simulink model "position"  (R2016b)
settings: Solver=VariableStepAuto  StartTime=0.0  StopTime=1  RelTol=1e-3
model workspace (MAT data in the model file):
  TL = 0
  Ti = 0.001
  fpwm = 5000
  ts = 5e-06
undefined symbols (not defined in the file): Kii, Kiw, Kpi, Kpw, pmsm, Ts, Tw
libraries: nesl_utility x13, fl_lib x10, simulink x6, pe_lib x4, pePwmGeneratorTwoLevel x1
settings Model: Creator=25097  LastModifiedBy=25097

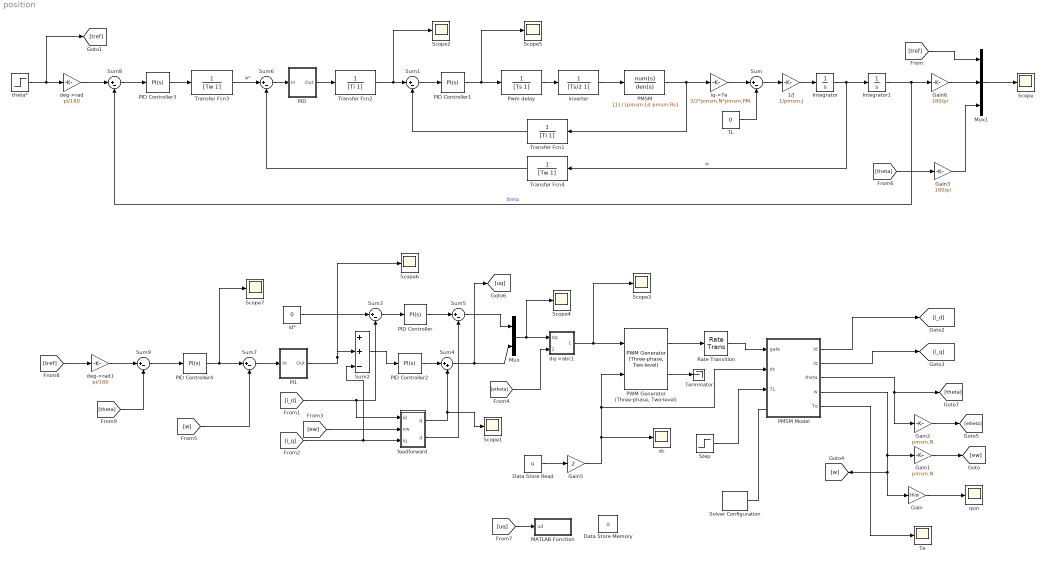
== system position ==
  1/J : Gain  Gain=1/pmsm.J
  Data Store Memory : DataStoreMemory  DataStoreName=u  ReadBeforeWriteMsg=warning  WriteAfterWriteMsg=warning  WriteAfterReadMsg=warning  InitialValue=10  ShowAdditionalParam=off  OutDataTypeStr=double
  Data Store Read : DataStoreRead  DataStoreName=u  DataStoreElements=u
  Gain : Gain  Gain=30/pi
  Gain1 : Gain  Gain=pmsm.N
  Gain2 : Gain  Gain=pmsm.N
  Gain3 : Gain  Gain=180/pi
  Gain5 : Gain  Gain=2
  Gain6 : Gain  Gain=180/pi
  Integrator : Integrator
  Integrator1 : Integrator
  MATLAB Function : MATLAB Function  TreatAsAtomicUnit=on
  Mux : Mux  Inputs=2
  Mux1 : Mux  Inputs=3
  PI1 : Subsystem
  PID : Subsystem
  PID Controller : simulink/Continuous/PID Controller  Controller=PI  TimeDomain=Continuous-time  SampleTime=-1  IntegratorMethod=Forward Euler  FilterMethod=Forward Euler  Form=Parallel  UseFilter=on  ControllerParametersSource=internal  P=Kpi  I=Kii  D=0  N=100  InitialConditionSource=internal  InitialConditionForIntegrator=0  InitialConditionForFilter=0  ExternalReset=none  LimitOutput=off  UpperSaturationLimit=inf  LowerSaturationLimit=-inf  LinearizeAsGain=on  AntiWindupMode=none  Kb=1  TrackingMode=off  Kt=1  PParamMin=[]  PParamMax=[]  IParamMin=[]  IParamMax=[]  DParamMin=[]  DParamMax=[]  NParamMin=[]  NParamMax=[]  KbParamMin=[]  KbParamMax=[]  KtParamMin=[]  KtParamMax=[]  POutMin=[]  POutMax=[]  IOutMin=[]  IOutMax=[]  DOutMin=[]  DOutMax=[]  NOutMin=[]  NOutMax=[]  KbOutMin=[]  KbOutMax=[]  KtOutMin=[]  KtOutMax=[]  IntegratorOutMin=[]  IntegratorOutMax=[]  FilterOutMin=[]  FilterOutMax=[]  SumOutMin=[]  SumOutMax=[]  SumI1OutMin=[]  SumI1OutMax=[]  SumI2OutMin=[]  SumI2OutMax=[]  SumI3OutMin=[]  SumI3OutMax=[]  SumDOutMin=[]  SumDOutMax=[]  SaturationOutMin=[]  SaturationOutMax=[]  IntegratorContinuousStateAttributes=''  IntegratorStateMustResolveToSignalObject=off  IntegratorRTWStateStorageClass=Auto  FilterContinuousStateAttributes=''  FilterStateMustResolveToSignalObject=off  FilterRTWStateStorageClass=Auto  DifferentiatorICPrevScaledInput=0  DifferentiatorOutMin=[]  DifferentiatorOutMax=[]
  PID Controller1 : simulink/Continuous/PID Controller  Controller=PI  TimeDomain=Continuous-time  SampleTime=-1  IntegratorMethod=Forward Euler  FilterMethod=Forward Euler  Form=Parallel  UseFilter=on  ControllerParametersSource=internal  P=Kpi  I=Kii  D=0  N=100  InitialConditionSource=internal  InitialConditionForIntegrator=0  InitialConditionForFilter=0  ExternalReset=none  LimitOutput=off  UpperSaturationLimit=5  LowerSaturationLimit=-5  LinearizeAsGain=on  AntiWindupMode=none  Kb=1  TrackingMode=off  Kt=1  PParamMin=[]  PParamMax=[]  IParamMin=[]  IParamMax=[]  DParamMin=[]  DParamMax=[]  NParamMin=[]  NParamMax=[]  KbParamMin=[]  KbParamMax=[]  KtParamMin=[]  KtParamMax=[]  POutMin=[]  POutMax=[]  IOutMin=[]  IOutMax=[]  DOutMin=[]  DOutMax=[]  NOutMin=[]  NOutMax=[]  KbOutMin=[]  KbOutMax=[]  KtOutMin=[]  KtOutMax=[]  IntegratorOutMin=[]  IntegratorOutMax=[]  FilterOutMin=[]  FilterOutMax=[]  SumOutMin=[]  SumOutMax=[]  SumI1OutMin=[]  SumI1OutMax=[]  SumI2OutMin=[]  SumI2OutMax=[]  SumI3OutMin=[]  SumI3OutMax=[]  SumDOutMin=[]  SumDOutMax=[]  SaturationOutMin=[]  SaturationOutMax=[]  IntegratorContinuousStateAttributes=''  IntegratorStateMustResolveToSignalObject=off  IntegratorRTWStateStorageClass=Auto  FilterContinuousStateAttributes=''  FilterStateMustResolveToSignalObject=off  FilterRTWStateStorageClass=Auto  DifferentiatorICPrevScaledInput=0  DifferentiatorOutMin=[]  DifferentiatorOutMax=[]
  PID Controller2 : simulink/Continuous/PID Controller  Controller=PI  TimeDomain=Continuous-time  SampleTime=-1  IntegratorMethod=Forward Euler  FilterMethod=Forward Euler  Form=Parallel  UseFilter=on  ControllerParametersSource=internal  P=Kpi  I=Kii  D=0  N=100  InitialConditionSource=internal  InitialConditionForIntegrator=0  InitialConditionForFilter=0  ExternalReset=none  LimitOutput=off  UpperSaturationLimit=inf  LowerSaturationLimit=-inf  LinearizeAsGain=on  AntiWindupMode=none  Kb=1  TrackingMode=off  Kt=1  PParamMin=[]  PParamMax=[]  IParamMin=[]  IParamMax=[]  DParamMin=[]  DParamMax=[]  NParamMin=[]  NParamMax=[]  KbParamMin=[]  KbParamMax=[]  KtParamMin=[]  KtParamMax=[]  POutMin=[]  POutMax=[]  IOutMin=[]  IOutMax=[]  DOutMin=[]  DOutMax=[]  NOutMin=[]  NOutMax=[]  KbOutMin=[]  KbOutMax=[]  KtOutMin=[]  KtOutMax=[]  IntegratorOutMin=[]  IntegratorOutMax=[]  FilterOutMin=[]  FilterOutMax=[]  SumOutMin=[]  SumOutMax=[]  SumI1OutMin=[]  SumI1OutMax=[]  SumI2OutMin=[]  SumI2OutMax=[]  SumI3OutMin=[]  SumI3OutMax=[]  SumDOutMin=[]  SumDOutMax=[]  SaturationOutMin=[]  SaturationOutMax=[]  IntegratorContinuousStateAttributes=''  IntegratorStateMustResolveToSignalObject=off  IntegratorRTWStateStorageClass=Auto  FilterContinuousStateAttributes=''  FilterStateMustResolveToSignalObject=off  FilterRTWStateStorageClass=Auto  DifferentiatorICPrevScaledInput=0  DifferentiatorOutMin=[]  DifferentiatorOutMax=[]
  PID Controller3 : simulink/Continuous/PID Controller  Controller=PI  TimeDomain=Continuous-time  SampleTime=-1  IntegratorMethod=Forward Euler  FilterMethod=Forward Euler  Form=Parallel  UseFilter=on  ControllerParametersSource=internal  P=19  I=8.8  D=0  N=100  InitialConditionSource=internal  InitialConditionForIntegrator=0  InitialConditionForFilter=0  ExternalReset=none  LimitOutput=off  UpperSaturationLimit=inf  LowerSaturationLimit=-inf  LinearizeAsGain=on  AntiWindupMode=none  Kb=1  TrackingMode=off  Kt=1  PParamMin=[]  PParamMax=[]  IParamMin=[]  IParamMax=[]  DParamMin=[]  DParamMax=[]  NParamMin=[]  NParamMax=[]  KbParamMin=[]  KbParamMax=[]  KtParamMin=[]  KtParamMax=[]  POutMin=[]  POutMax=[]  IOutMin=[]  IOutMax=[]  DOutMin=[]  DOutMax=[]  NOutMin=[]  NOutMax=[]  KbOutMin=[]  KbOutMax=[]  KtOutMin=[]  KtOutMax=[]  IntegratorOutMin=[]  IntegratorOutMax=[]  FilterOutMin=[]  FilterOutMax=[]  SumOutMin=[]  SumOutMax=[]  SumI1OutMin=[]  SumI1OutMax=[]  SumI2OutMin=[]  SumI2OutMax=[]  SumI3OutMin=[]  SumI3OutMax=[]  SumDOutMin=[]  SumDOutMax=[]  SaturationOutMin=[]  SaturationOutMax=[]  IntegratorContinuousStateAttributes=''  IntegratorStateMustResolveToSignalObject=off  IntegratorRTWStateStorageClass=Auto  FilterContinuousStateAttributes=''  FilterStateMustResolveToSignalObject=off  FilterRTWStateStorageClass=Auto  DifferentiatorICPrevScaledInput=0  DifferentiatorOutMin=[]  DifferentiatorOutMax=[]
  PID Controller4 : simulink/Continuous/PID Controller  Controller=PI  TimeDomain=Continuous-time  SampleTime=-1  IntegratorMethod=Forward Euler  FilterMethod=Forward Euler  Form=Parallel  UseFilter=on  ControllerParametersSource=internal  P=19  I=20  D=0  N=100  InitialConditionSource=internal  InitialConditionForIntegrator=0  InitialConditionForFilter=0  ExternalReset=none  LimitOutput=off  UpperSaturationLimit=inf  LowerSaturationLimit=-inf  LinearizeAsGain=on  AntiWindupMode=none  Kb=1  TrackingMode=off  Kt=1  PParamMin=[]  PParamMax=[]  IParamMin=[]  IParamMax=[]  DParamMin=[]  DParamMax=[]  NParamMin=[]  NParamMax=[]  KbParamMin=[]  KbParamMax=[]  KtParamMin=[]  KtParamMax=[]  POutMin=[]  POutMax=[]  IOutMin=[]  IOutMax=[]  DOutMin=[]  DOutMax=[]  NOutMin=[]  NOutMax=[]  KbOutMin=[]  KbOutMax=[]  KtOutMin=[]  KtOutMax=[]  IntegratorOutMin=[]  IntegratorOutMax=[]  FilterOutMin=[]  FilterOutMax=[]  SumOutMin=[]  SumOutMax=[]  SumI1OutMin=[]  SumI1OutMax=[]  SumI2OutMin=[]  SumI2OutMax=[]  SumI3OutMin=[]  SumI3OutMax=[]  SumDOutMin=[]  SumDOutMax=[]  SaturationOutMin=[]  SaturationOutMax=[]  IntegratorContinuousStateAttributes=''  IntegratorStateMustResolveToSignalObject=off  IntegratorRTWStateStorageClass=Auto  FilterContinuousStateAttributes=''  FilterStateMustResolveToSignalObject=off  FilterRTWStateStorageClass=Auto  DifferentiatorICPrevScaledInput=0  DifferentiatorOutMin=[]  DifferentiatorOutMax=[]
  "PMSM " : TransferFcn  Denominator=[pmsm.Ld pmsm.Rs]
  PMSM Model : Subsystem
      settings: MinAlgLoopOccurrences=on
  "PWM Generator (Three-phase, Two-level)" : pePwmGeneratorTwoLevel/PWM Generator (Three-phase, Two-level)  OverrideUsingVariant=NaturalMode  PWMMode=Continuous PWM (CPWM)  CPWMMode=SPWM: sinusoidal PWM  DPWMMode=60 DPWM: 60 degree discontinuous PWM  fsw=fpwm  Ts=ts
      settings: SamplingMode=Natural
  "Pwm delay " : TransferFcn  Denominator=[Ts 1]
  Rate Transition : RateTransition
  Scope{,1..7} (8 alike) : Scope
  Solver Configuration : nesl_utility/Solver Configuration  PhysicalDomain=network_engine_domain  SubClassName=solver  LeftPortType=input  RightPortType=generic  Accelerate=off  Tones=[]  Harmonics=[]  SimulateNoise=off  Profile=off  UseLocalSampling=off  EnableSwitchedLinearOptims=on  FrequencyDomain=off  UseCCode=off  RelTol=0.001  AbsTol=1e-06  MinStep=1e-09  ToWorkspace=off  RevertToSquareIcSolve=off  NumHomotopyIterations=100  PhasorMode=off  PhasorModeNumHarmonics=1  OverrideAbsTol=off  DoDC=off  ResidualTolerance=1e-07  UseLocalSolver=off  LocalSolverChoice=NE_BACKWARD_EULER_ADVANCER  LocalSolverSampleTime=1e-6  DoFixedCost=off  MaxNonlinIter=3  MaxModeIter=2  LinearAlgebra=Sparse  DelaysMemoryBudget=1024  AutomaticFiltering=on  FilteringTimeConstant=0.001
  Step : Step  Time=0.4  After=TL  SampleTime=0
  Sum{,1,3,5..9} (8 alike) : Sum  Inputs=|+-
  Sum2 : Sum  Inputs=|++-
  Sum4 : Sum  Inputs=|++
  TL : Constant  Value=0
  Te : Scope
  Terminator : Terminator
  Transfer Fcn1 : TransferFcn  Denominator=[Ti 1]
  Transfer Fcn2 : TransferFcn  Denominator=[Ti 1]
  Transfer Fcn3 : TransferFcn  Denominator=[Tw 1]
  Transfer Fcn4 : TransferFcn  Numerator=[ 1]  Denominator=[Tw 1]
  dc : Scope
  deg->rad : Gain  Gain=pi/180
  deg->rad1 : Gain  Gain=pi/180
  dq->abc1 : Subsystem
  "feedforward " : Subsystem
  id* : Constant  Value=0
  inverter : TransferFcn  Denominator=[Ts/2 1]
  iq->Te : Gain  Gain=3/2*pmsm.N*pmsm.PM
  rpm : Scope
  theta* : Step  Time=0.05  After=30  SampleTime=0
  wires:
  Transfer Fcn2/1 -> Scope2/1, Sum1/1
  Sum1/1 -> PID Controller1/1
  PID Controller1/1 -> Scope5/1, "Pwm delay "/1
  "Pwm delay "/1 -> inverter/1
  inverter/1 -> "PMSM "/1
  "PMSM "/1 -> Transfer Fcn1/1, iq->Te/1
  Transfer Fcn1/1 -> Sum1/2
  Sum2/1 -> PID Controller2/1
  PID Controller2/1 -> Sum4/1
  id*/1 -> Sum3/1
  Sum3/1 -> PID Controller/1
  PID Controller/1 -> Sum5/1
  "feedforward "/1(q) -> Sum4/2, Scope1/1
  "feedforward "/2(d) -> Sum5/2
  [ew] -> "feedforward "/2(ew)
  Sum4/1 -> [uq], Mux/2
  Sum5/1 -> Mux/1
  Mux/1 -> Scope4/1, dq->abc1/1(dq)
  [etheta] -> dq->abc1/2("theta ")
  Gain5/1 -> dc/1, "PWM Generator (Three-phase, Two-level)"/2, PMSM Model/2(dc)
  "PWM Generator (Three-phase, Two-level)"/2 -> Terminator/1
  PMSM Model/3(theta) -> Gain2/1, [theta]
  Mux1/1 -> Scope/1
  Gain/1 -> rpm/1
  PMSM Model/5("Te ") -> Te/1
  PMSM Model/4(w) -> Gain1/1, [w], Gain/1
  Gain2/1 -> [etheta]
  Gain1/1 -> [ew]
  PMSM Model/1(id) -> [i_d]
  PMSM Model/2(iq) -> [i_q]
  [i_d] -> "feedforward "/1("id "), Sum3/2
  [i_q] -> Sum2/3, "feedforward "/3(iq)
  dq->abc1/1(abc) -> Scope3/1, "PWM Generator (Three-phase, Two-level)"/1
  "PWM Generator (Three-phase, Two-level)"/1 -> Rate Transition/1
  Rate Transition/1 -> PMSM Model/1("gate ")
  iq->Te/1 -> Sum/1
  TL/1 -> Sum/2
  Sum/1 -> 1/J/1
  1/J/1 -> Integrator/1
  Integrator/1 -> Integrator1/1, Transfer Fcn4/1  "w"
  Transfer Fcn3/1 -> Sum6/1  "w*"
  Transfer Fcn4/1 -> Sum6/2
  PID Controller3/1 -> Transfer Fcn3/1
  Sum6/1 -> PID/1(In)
  PID/1(Out) -> Transfer Fcn2/1
  theta*/1 -> [tref], deg->rad/1
  Sum7/1 -> PI1/1(In)
  PI1/1(Out) -> Scope6/1, Sum2/2
  [w] -> Sum7/2
  [uq] -> MATLAB Function/1(ud)
  Data Store Read/1 -> Gain5/1
  Step/1 -> PMSM Model/3(TL)
  Integrator1/1 -> Sum8/2, Gain6/1  "theta"
  Gain6/1 -> Mux1/2
  deg->rad/1 -> Sum8/1
  Sum8/1 -> PID Controller3/1
  [tref] -> Mux1/1
  PID Controller4/1 -> Scope7/1, Sum7/1
  [tref] -> deg->rad1/1
  deg->rad1/1 -> Sum9/1
  Sum9/1 -> PID Controller4/1
  [theta] -> Sum9/2
  [theta] -> Gain3/1
  Gain3/1 -> Mux1/3
  connections:
  Solver Configuration/RConn1 -- PMSM Model/LConn1

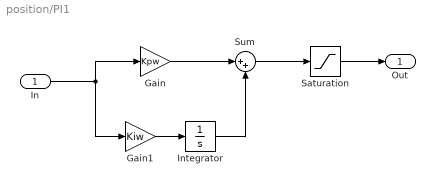
== system position/PI1 ==
  In : Inport
  Gain : Gain  Gain=Kpw
  Gain1 : Gain  Gain=Kiw
  Integrator : Integrator  LimitOutput=on  UpperSaturationLimit=pmsm.Imax*0.5  LowerSaturationLimit=-pmsm.Imax*0.5
  Saturation : Saturate  UpperLimit=pmsm.Imax  LowerLimit=-pmsm.Imax
  Sum : Sum  Inputs=|++
  Out : Outport
  wires:
  Saturation/1 -> Out/1
  Sum/1 -> Saturation/1
  Integrator/1 -> Sum/2
  Gain/1 -> Sum/1
  Gain1/1 -> Integrator/1
  In/1 -> Gain/1, Gain1/1

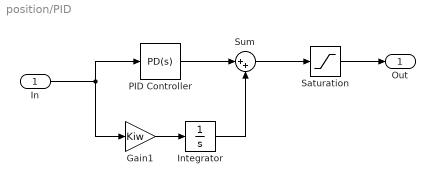
== system position/PID ==
  In : Inport
  Gain1 : Gain  Gain=Kiw
  Integrator : Integrator  LimitOutput=on  UpperSaturationLimit=pmsm.Imax*0.5  LowerSaturationLimit=-pmsm.Imax*0.5
  PID Controller : simulink/Continuous/PID Controller  Controller=PD  TimeDomain=Continuous-time  SampleTime=-1  IntegratorMethod=Forward Euler  FilterMethod=Forward Euler  Form=Parallel  UseFilter=on  ControllerParametersSource=internal  P=Kpw  I=1  D=0.01  N=100  InitialConditionSource=internal  InitialConditionForIntegrator=0  InitialConditionForFilter=0  ExternalReset=none  LimitOutput=off  UpperSaturationLimit=inf  LowerSaturationLimit=-inf  LinearizeAsGain=on  AntiWindupMode=none  Kb=1  TrackingMode=off  Kt=1  PParamMin=[]  PParamMax=[]  IParamMin=[]  IParamMax=[]  DParamMin=[]  DParamMax=[]  NParamMin=[]  NParamMax=[]  KbParamMin=[]  KbParamMax=[]  KtParamMin=[]  KtParamMax=[]  POutMin=[]  POutMax=[]  IOutMin=[]  IOutMax=[]  DOutMin=[]  DOutMax=[]  NOutMin=[]  NOutMax=[]  KbOutMin=[]  KbOutMax=[]  KtOutMin=[]  KtOutMax=[]  IntegratorOutMin=[]  IntegratorOutMax=[]  FilterOutMin=[]  FilterOutMax=[]  SumOutMin=[]  SumOutMax=[]  SumI1OutMin=[]  SumI1OutMax=[]  SumI2OutMin=[]  SumI2OutMax=[]  SumI3OutMin=[]  SumI3OutMax=[]  SumDOutMin=[]  SumDOutMax=[]  SaturationOutMin=[]  SaturationOutMax=[]  IntegratorContinuousStateAttributes=''  IntegratorStateMustResolveToSignalObject=off  IntegratorRTWStateStorageClass=Auto  FilterContinuousStateAttributes=''  FilterStateMustResolveToSignalObject=off  FilterRTWStateStorageClass=Auto  DifferentiatorICPrevScaledInput=0  DifferentiatorOutMin=[]  DifferentiatorOutMax=[]
  Saturation : Saturate  UpperLimit=pmsm.Imax  LowerLimit=-pmsm.Imax
  Sum : Sum  Inputs=|++
  Out : Outport
  wires:
  In/1 -> PID Controller/1, Gain1/1
  Gain1/1 -> Integrator/1
  PID Controller/1 -> Sum/1
  Integrator/1 -> Sum/2
  Sum/1 -> Saturation/1
  Saturation/1 -> Out/1

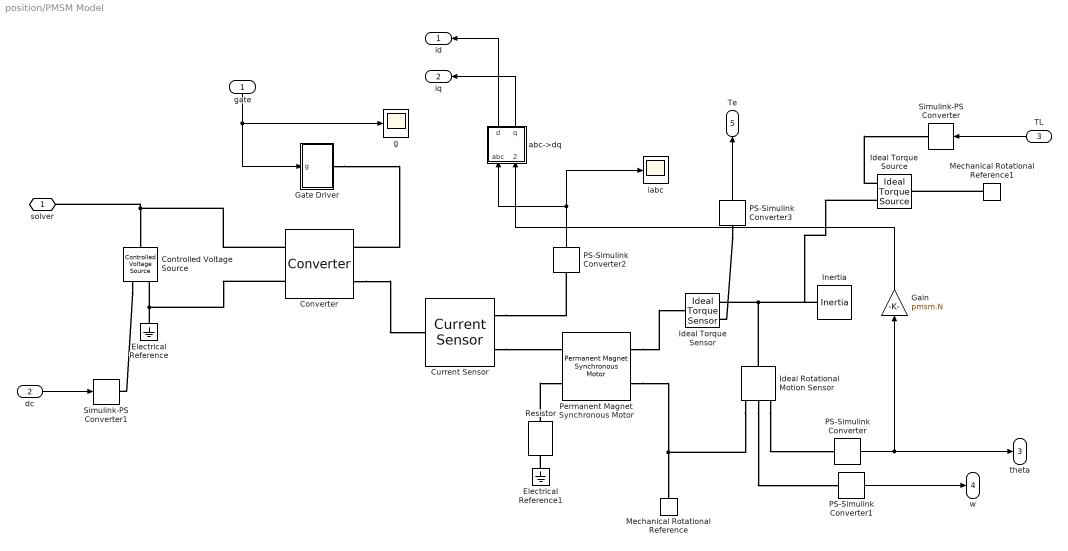
== system position/PMSM Model ==
  "gate " : Inport
  dc : Inport  Port=2
  TL : Inport  Port=3
  Controlled Voltage Source : fl_lib/Electrical/Electrical Sources/Controlled Voltage Source
  Converter : pe_lib/Semiconductors/Converter  device_type=2  Vf=0.8 V  Ron=0.001 Ohm  Rds=0.001 Ohm  Goff=1e-8 1/Ohm  Vth=0.5 V  Vgt=1 V  Vgt_off=-1 V  Ih=1 A  diode_param=1  diode_Vf=0.8 V  diode_Ron=0.001 Ohm  diode_Goff=1e-5 1/Ohm  diode_C=50 nF  diode_iRM=-235 A  diode_iF=300 A  diode_idot=-50 A/us  diode_trr_param=1  diode_trr_factor=3  diode_trr=15 us  diode_Qrr=1.5e+3 s*uA  snubber_type=0  Rs=0.1 Ohm  Cs=1e-7 F
  Current Sensor : pe_lib/Sensors/Current Sensor
  Electrical Reference : fl_lib/Electrical/Electrical Elements/Electrical Reference
  Electrical Reference1 : fl_lib/Electrical/Electrical Elements/Electrical Reference
  Gain : Gain  Gain=pmsm.N
  Gate Driver : Subsystem
  Ideal Rotational Motion Sensor : fl_lib/Mechanical/Mechanical Sensors/Ideal Rotational Motion Sensor  offset=0 rad
  Ideal Torque Sensor : fl_lib/Mechanical/Mechanical Sensors/Ideal Torque Sensor
  Ideal Torque Source : fl_lib/Mechanical/Mechanical Sources/Ideal Torque Source
  Inertia : fl_lib/Mechanical/Rotational Elements/Inertia  inertia=pmsm.J kg*m^2  w_specify=off  w_priority=High  w=0 rad/s  t_specify=off  t_priority=None  t=0 N*m
  Mechanical Rotational Reference : fl_lib/Mechanical/Rotational Elements/Mechanical Rotational Reference
  Mechanical Rotational Reference1 : fl_lib/Mechanical/Rotational Elements/Mechanical Rotational Reference
  PS-Simulink Converter{,1..3} (4 alike) : nesl_utility/PS-Simulink Converter  PhysicalDomain=network_engine_domain  SubClassName=ps_output  LeftPortType=input  RightPortType=output  PseudoPeriodic=off  Frequencies=[]  Unit=1  AffineConversion=off
  Permanent Magnet Synchronous Motor : pe_lib/Machines/Permanent Magnet Rotor/Permanent Magnet Synchronous Motor  nPolePairs=pmsm.N  pm_flux_linkage=pmsm.PM Wb  stator_param=1  Ld=pmsm.Ld H  Lq=pmsm.Ld H  L0=pmsm.Ld H  Ls=0.0002 H  Lm=0.00002 H  Ms=0.00002 H  Rs=pmsm.Rs Ohm  initial_currents=[0.0, 0.0, 0.0] A  axes_param=2  angular_position0=0 rad  rotor_offset=-pi / 2 rad  shift_3ph=[nan, nan, nan] rad  sqrt2OverSqrt3=nan  oneOverSqrt2=nan  twoPiOver3=nan  Lmin=1e-9 H
  Resistor : fl_lib/Electrical/Electrical Elements/Resistor  R=1e9 Ohm  i_specify=off  i_priority=None  i=0 A  v_specify=off  v_priority=None  v=0 V
  Simulink-PS Converter : nesl_utility/Simulink-PS Converter  PhysicalDomain=network_engine_domain  SubClassName=ps_input  LeftPortType=input  RightPortType=output  PseudoPeriodic=off  Frequencies=[]  NoiseDistribution=none  NoiseParameters=[]  Unit=1  AffineConversion=off  InputFiltering=off  SimscapeFilterOrder=1  InputFilterTimeConstant=0.001  UdotUserProvided=1
  Simulink-PS Converter1 : nesl_utility/Simulink-PS Converter  PhysicalDomain=network_engine_domain  SubClassName=ps_input  LeftPortType=input  RightPortType=output  PseudoPeriodic=off  Frequencies=[]  NoiseDistribution=none  NoiseParameters=[]  Unit=1  AffineConversion=off  InputFiltering=off  SimscapeFilterOrder=1  InputFilterTimeConstant=0.001  UdotUserProvided=1
  abc->dq : Subsystem
  g : Scope
  iabc : Scope
  "solver " : PMIOPort  Port=1  Side=Left
  id : Outport
  iq : Outport  Port=2
  theta : Outport  Port=3
  w : Outport  Port=4
  "Te " : Outport  Port=5
  wires:
  PS-Simulink Converter/1 -> Gain/1, theta/1
  PS-Simulink Converter2/1 -> abc->dq/1(abc), iabc/1
  PS-Simulink Converter1/1 -> w/1
  abc->dq/1(d) -> id/1
  abc->dq/2(q) -> iq/1
  PS-Simulink Converter3/1 -> "Te "/1
  Gain/1 -> abc->dq/2(theta)
  "gate "/1 -> g/1, Gate Driver/1(g)
  dc/1 -> Simulink-PS Converter1/1
  TL/1 -> Simulink-PS Converter/1
  connections:
  Electrical Reference/LConn1 -- Converter/RConn2 -- Controlled Voltage Source/RConn2
  Converter/RConn1 -- Controlled Voltage Source/LConn1 -- "solver "/RConn1
  Current Sensor/RConn1 -- PS-Simulink Converter2/LConn1
  Converter/LConn2 -- Current Sensor/LConn1
  Resistor/LConn1 -- Permanent Magnet Synchronous Motor/LConn2
  Current Sensor/RConn2 -- Permanent Magnet Synchronous Motor/LConn1
  Electrical Reference1/LConn1 -- Resistor/RConn1
  Gate Driver/RConn1 -- Converter/LConn1
  Permanent Magnet Synchronous Motor/RConn2 -- Mechanical Rotational Reference/LConn1 -- Ideal Rotational Motion Sensor/RConn1
  Permanent Magnet Synchronous Motor/RConn1 -- Ideal Torque Sensor/LConn1
  Ideal Rotational Motion Sensor/LConn1 -- Ideal Torque Sensor/RConn1 -- Ideal Torque Source/RConn2 -- Inertia/LConn1
  Ideal Rotational Motion Sensor/RConn3 -- PS-Simulink Converter/LConn1
  Ideal Rotational Motion Sensor/RConn2 -- PS-Simulink Converter1/LConn1
  PS-Simulink Converter3/LConn1 -- Ideal Torque Sensor/RConn2
  Controlled Voltage Source/RConn1 -- Simulink-PS Converter1/RConn1
  Mechanical Rotational Reference1/LConn1 -- Ideal Torque Source/LConn1
  Ideal Torque Source/RConn1 -- Simulink-PS Converter/RConn1

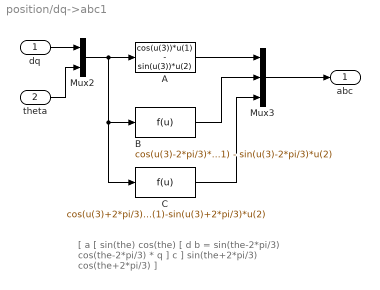
== system position/dq->abc1 ==
  note: [ a        [  sin(the)               cos(the)                 [ d
      |
      |   b    =     sin(the-2*pi/3)    cos(the-2*pi/3)    *    q ]
      |
      |   c ]         sin(the+2*pi/3)   cos(the+2*pi/3) ]
  dq : Inport
  "theta " : Inport  Port=2
  A : Fcn  Expr=cos(u(3))*u(1) - sin(u(3))*u(2)
  B : Fcn  Expr=cos(u(3)-2*pi/3)*u(1) - sin(u(3)-2*pi/3)*u(2)
  C : Fcn  Expr=cos(u(3)+2*pi/3)*u(1)-sin(u(3)+2*pi/3)*u(2)
  Mux2 : Mux  Inputs=2
  Mux3 : Mux  Inputs=3
  abc : Outport
  wires:
  Mux3/1 -> abc/1
  C/1 -> Mux3/3
  A/1 -> Mux3/1
  dq/1 -> Mux2/1
  "theta "/1 -> Mux2/2
  Mux2/1 -> C/1, B/1, A/1
  B/1 -> Mux3/2

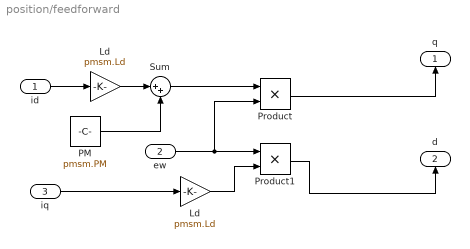
== system position/feedforward  ==
  "id " : Inport
  ew : Inport  Port=2
  iq : Inport  Port=3
  Ld : Gain  Gain=pmsm.Ld
  "Ld " : Gain  Gain=pmsm.Ld
  PM : Constant  Value=pmsm.PM
  Product : Product
  Product1 : Product
  Sum : Sum  Inputs=|++
  q : Outport
  d : Outport  Port=2
  wires:
  "id "/1 -> Ld/1
  PM/1 -> Sum/2
  Ld/1 -> Sum/1
  "Ld "/1 -> Product1/2
  Product/1 -> q/1
  Sum/1 -> Product/1
  Product1/1 -> d/1
  iq/1 -> "Ld "/1
  ew/1 -> Product1/1, Product/2

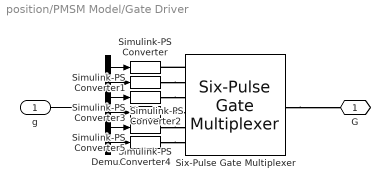
== system position/PMSM Model/Gate Driver ==
  g : Inport
  Demux : Demux  Outputs=6
  Simulink-PS Converter{,1..5} (6 alike) : nesl_utility/Simulink-PS Converter  PhysicalDomain=network_engine_domain  SubClassName=ps_input  LeftPortType=input  RightPortType=output  PseudoPeriodic=off  Frequencies=[]  NoiseDistribution=none  NoiseParameters=[]  Unit=1  AffineConversion=off  InputFiltering=off  SimscapeFilterOrder=1  InputFilterTimeConstant=0.001  UdotUserProvided=1
  Six-Pulse Gate Multiplexer : pe_lib/Semiconductors/Six-Pulse Gate Multiplexer  R=0 Ohm
  G : PMIOPort  Port=1  Side=Right
  wires:
  g/1 -> Demux/1
  Demux/1 -> Simulink-PS Converter/1
  Demux/2 -> Simulink-PS Converter1/1
  Demux/3 -> Simulink-PS Converter2/1
  Demux/4 -> Simulink-PS Converter3/1
  Demux/5 -> Simulink-PS Converter4/1
  Demux/6 -> Simulink-PS Converter5/1
  connections:
  Six-Pulse Gate Multiplexer/LConn1 -- Simulink-PS Converter/RConn1
  Simulink-PS Converter1/RConn1 -- Six-Pulse Gate Multiplexer/LConn2
  Simulink-PS Converter2/RConn1 -- Six-Pulse Gate Multiplexer/LConn3
  Simulink-PS Converter3/RConn1 -- Six-Pulse Gate Multiplexer/LConn4
  Simulink-PS Converter4/RConn1 -- Six-Pulse Gate Multiplexer/LConn5
  Simulink-PS Converter5/RConn1 -- Six-Pulse Gate Multiplexer/LConn6
  Six-Pulse Gate Multiplexer/RConn1 -- G/RConn1

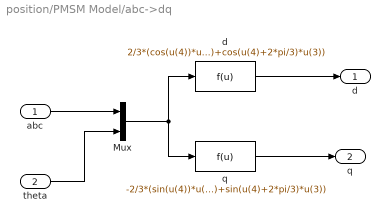
== system position/PMSM Model/abc->dq ==
  abc : Inport
  theta : Inport  Port=2
  Mux : Mux  Inputs=2
  "d " : Fcn  Expr=2/3*(cos(u(4))*u(1)+cos(u(4)-2*pi/3)*u(2)+cos(u(4)+2*pi/3)*u(3))
  "q " : Fcn  Expr=-2/3*(sin(u(4))*u(1)+sin(u(4)-2*pi/3)*u(2)+sin(u(4)+2*pi/3)*u(3))
  d : Outport
  q : Outport  Port=2
  wires:
  "d "/1 -> d/1
  "q "/1 -> q/1
  abc/1 -> Mux/1
  Mux/1 -> "q "/1, "d "/1
  theta/1 -> Mux/2

== matlab function position/MATLAB Function ==
  data: ud input; u data_store_memory
function fcn(ud)
global u;
if ud < 8
    u = 10;
else
    if ud > 0.9 * u
        u = u/0.9;
    else if ud < 0.7 * u
        u = u*0.7;
        end
    end

end
